simulink library "Lib_PFSys_GenericMotor_TMATS"  (R2018a)
settings: Solver=ode45  StartTime=0.0  StopTime=10.0  RelTol=1e-3  EnableMultiTasking=on
libraries: Lib_PF_BusLoadDC_TMATS x1, Lib_PF_LineDC_TMATS x1
Description:
  | Thomas Modules
settings Model: Creator=jwchapm2  LastModifiedBy=mebell
settings DataIOCC: LimitDataPoints=on  SaveFormat=Array
settings OptimizationCC: ExpressionDepthLimit=2147483647  LifeSpan=inf
settings DebuggingCC: UnderspecifiedInitializationDetection=Classic  MergeDetectMultiDrivingBlocksExec=none  SolverPrmCheckMsg=warning  StateNameClashWarn=warning  SFUnexpectedBacktrackingDiag=warning  SFNoUnconditionalDefaultTransitionDiag=warning  SFExecutionAtInitializationDiag=none
settings HardwareCC: ProdBitPerPointer=32  ProdBitPerSizeT=32  ProdBitPerPtrDiffT=32  ProdLargestAtomicFloat=None  ProdIntDivRoundTo=Undefined  ProdEndianess=Unspecified  ProdWordSize=32  ProdHWDeviceType=32-bit Generic
settings ModelReferenceCC: PropagateSignalLabelsOutOfModel=off
settings CodeAppCC: StateflowObjectComments=on
settings GRTTargetCC: TargetLangStandard=C89/C90 (ANSI)  GeneratePreprocessorConditionals=Disable all
settings ConfigComp: CovMetricSettings=dw  CovHtmlReporting=on  CovSaveCumulativeToWorkspaceVar=on  CovSaveSingleToWorkspaceVar=on  CovExternalEMLEnable=off

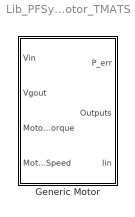
== system Lib_PFSys_GenericMotor_TMATS ==
  Generic Motor : Subsystem  mask(Motor){X_C_SpeedVec_M=[0.0 0.1 1.0], Y_C_TorqueVec_M=[0.0 0.1 1.0], T_C_EffArray_M=[0.5 0.5 0.5; 0.5 1.0 1.0; 0.5 1.0 1.0], Z_M=0.01}
      mask prompts: X_C_SpeedVec_M "X_C_SpeedVec_M - Efficiency Table Speed Vector (X-axis)(nx1)"; Y_C_TorqueVec_M "Y_C_TorqueVec_M - Efficiency Table Torque Vector (Y-axis)(mx1)"; T_C_EffArray_M "T_C_EffArray_M - Efficiency Table Values (Eff = f(i, V)(nxm)"; Z_M "Z_M - Resistive Impedance"
      mask help:
      | This block represents a generic motor with a purely resistive input
      | impedance, and a lumped efficiency/loss model, specified as a lookup table.

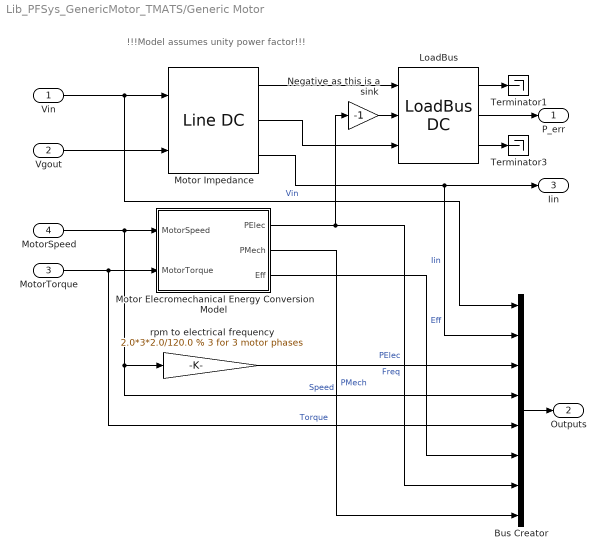
== system Lib_PFSys_GenericMotor_TMATS/Generic Motor ==
  note: !!!Model assumes unity power factor!!!
  Vin : Inport
  Vgout : Inport  Port=2
  MotorTorque : Inport  Port=3
  MotorSpeed : Inport  Port=4
  Bus Creator : BusCreator  Inputs=8
  LoadBus : Lib_PF_BusLoadDC_TMATS/LoadBus DC  PeInEN_M=on  P_M=-2  BlkNm_M=double(gcb)
  Motor Elecromechanical Energy Conversion Model : Subsystem
  Motor Impedance : Lib_PF_LineDC_TMATS/Line DC  R_M=Z_M
  Negative as this is a sink : Gain  Gain=-1
  Terminator1 : Terminator
  Terminator3 : Terminator
  rpm to electrical frequency : Gain  Gain=2.0*3*2.0/120.0 % 3 for 3 motor phases
  P_err : Outport
  Outputs : Outport  Port=2
  Iin : Outport  Port=3
  wires:
  Motor Elecromechanical Energy Conversion Model/1(PElec) -> Negative as this is a sink/1, Bus Creator/7  "PElec"
  Negative as this is a sink/1 -> LoadBus/2
  Motor Impedance/2 -> LoadBus/3
  Motor Impedance/3 -> Iin/1, Bus Creator/2  "Iin"
  Motor Impedance/1 -> LoadBus/1
  Vgout/1 -> Motor Impedance/2
  Bus Creator/1 -> Outputs/1
  rpm to electrical frequency/1 -> Bus Creator/3  "Freq"
  MotorTorque/1 -> Bus Creator/5, Motor Elecromechanical Energy Conversion Model/2(MotorTorque)  "Torque"
  MotorSpeed/1 -> Motor Elecromechanical Energy Conversion Model/1(MotorSpeed), Bus Creator/4, rpm to electrical frequency/1  "Speed"
  LoadBus/3 -> Terminator3/1
  Vin/1 -> Bus Creator/1, Motor Impedance/1  "Vin"
  LoadBus/2 -> P_err/1
  LoadBus/1 -> Terminator1/1
  Motor Elecromechanical Energy Conversion Model/3(Eff) -> Bus Creator/6  "Eff"
  Motor Elecromechanical Energy Conversion Model/2(PMech) -> Bus Creator/8  "PMech"

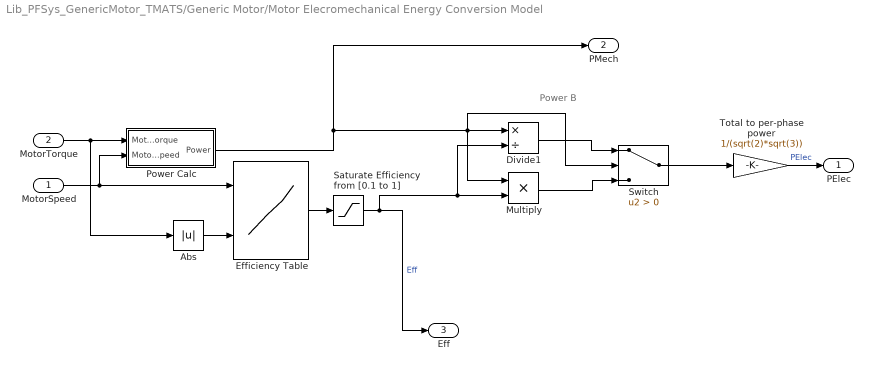
== system Lib_PFSys_GenericMotor_TMATS/Generic Motor/Motor Elecromechanical Energy Conversion Model ==
  note: Power B
  MotorSpeed : Inport
  MotorTorque : Inport  Port=2
  Abs : Abs
  Divide1 : Product  Inputs=*/
  Efficiency Table : Lookup_n-D  BreakpointsForDimension1=X_C_SpeedVec_M  BreakpointsForDimension2=Y_C_TorqueVec_M  Table=T_C_EffArray_M  ExtrapMethod=Clip  InternalRulePriority=Speed  RndMeth=Simplest  InputSameDT=on
  Multiply : Product
  Power Calc : Subsystem
  Saturate Efficiency from [0.1 to 1] : Saturate  UpperLimit=1  LowerLimit=0.1
  Switch : Switch  Criteria=u2 > Threshold
  Total to per-phase power : Gain  Gain=1/(sqrt(2)*sqrt(3))
  PElec : Outport
  PMech : Outport  Port=2
  Eff : Outport  Port=3
  wires:
  Efficiency Table/1 -> Saturate Efficiency from [0.1 to 1]/1
  Saturate Efficiency from [0.1 to 1]/1 -> Divide1/2, Multiply/2, Eff/1  "Eff"
  Abs/1 -> Efficiency Table/2
  Total to per-phase power/1 -> PElec/1  "PElec"
  MotorTorque/1 -> Abs/1, Power Calc/1(MotorTorque)
  MotorSpeed/1 -> Power Calc/2(MotorSpeed), Efficiency Table/1
  Power Calc/1(Power) -> Switch/2, Multiply/1, Divide1/1, PMech/1
  Divide1/1 -> Switch/1
  Multiply/1 -> Switch/3
  Switch/1 -> Total to per-phase power/1

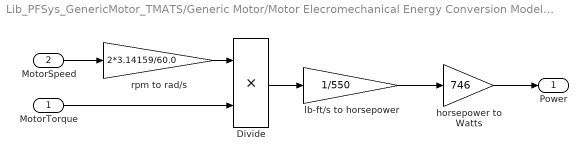
== system Lib_PFSys_GenericMotor_TMATS/Generic Motor/Motor Elecromechanical Energy Conversion Model/Power Calc ==
  MotorTorque : Inport
  MotorSpeed : Inport  Port=2
  Divide : Product  Inputs=**
  horsepower to Watts : Gain  Gain=746
  lb-ft/s to horsepower : Gain  Gain=1/550
  rpm to rad/s : Gain  Gain=2*3.14159/60.0
  Power : Outport
  wires:
  MotorSpeed/1 -> rpm to rad/s/1
  Divide/1 -> lb-ft/s to horsepower/1
  lb-ft/s to horsepower/1 -> horsepower to Watts/1
  MotorTorque/1 -> Divide/2
  rpm to rad/s/1 -> Divide/1
  horsepower to Watts/1 -> Power/1
